simulink model "lab03"  (R2024b)
settings: Solver=VariableStepAuto  StartTime=0.0  StopTime=1  MaxStep=0.001  RelTol=1e-3
values from neighbouring files (symbols this model uses):
  K = 19.4    [untitled.m]
  K_d = 0.0317    [untitled.m]
  K_r = 1.0309    [untitled.m]
  omega_end = 1    [untitled.m]
  tau_end = 0    [untitled.m]
settings Model: Creator=blji2  LastModifiedBy=blji2

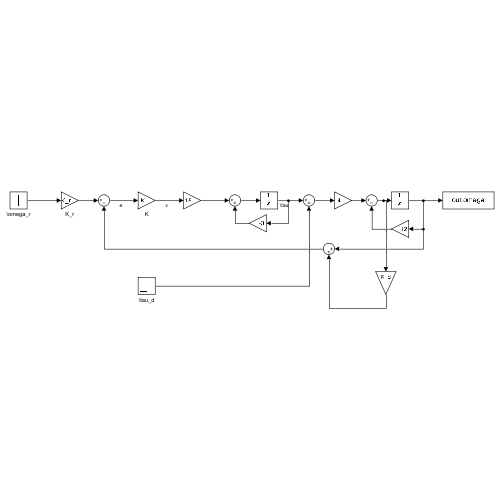
[thumbnail: Simulink's stored preview of the top-level diagram]
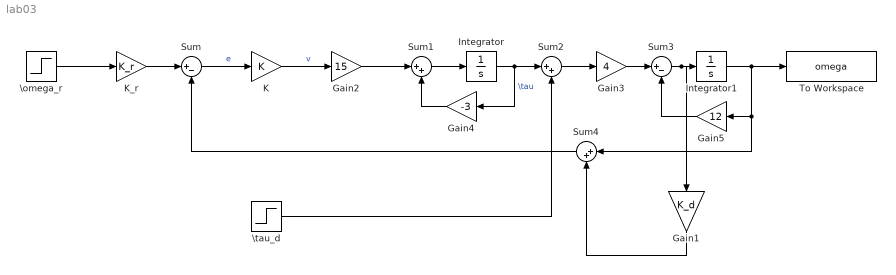
== system lab03 ==
  Gain1 : Gain  Gain=K_d
  Gain2 : Gain  Gain=15
  Gain3 : Gain  Gain=4
  Gain4 : Gain  Gain=-3
  Gain5 : Gain  Gain=12
  Integrator : Integrator
  Integrator1 : Integrator
  K : Gain  Gain=K
  K_r : Gain  Gain=K_r
  Sum : Sum  Inputs=|+-
  Sum1 : Sum  Inputs=|++
  Sum2 : Sum  Inputs=|++
  Sum3 : Sum  Inputs=|+-
  Sum4 : Sum  Inputs=|++
  To Workspace : ToWorkspace  VariableName=omega  SampleTime=-1
  \omega_r : Step  Time=0  After=omega_end  SampleTime=0
  \tau_d : Step  Time=0  After=tau_end  SampleTime=0
  wires:
  Sum1/1 -> Integrator/1
  Sum2/1 -> Gain3/1
  Integrator1/1 -> Sum4/1, Gain5/1, To Workspace/1
  Integrator/1 -> Gain4/1, Sum2/1  "\\tau"
  Gain2/1 -> Sum1/1
  K/1 -> Gain2/1  "v"
  Sum/1 -> K/1  "e"
  K_r/1 -> Sum/1
  \omega_r/1 -> K_r/1
  Gain4/1 -> Sum1/2
  Gain3/1 -> Sum3/1
  Sum3/1 -> Gain1/1, Integrator1/1
  Gain5/1 -> Sum3/2
  \tau_d/1 -> Sum2/2
  Sum4/1 -> Sum/2
  Gain1/1 -> Sum4/2
